simulink model "otwartaPetla"  (R2022b)
settings: Solver=VariableStepAuto  StartTime=0.0  StopTime=10.0  RelTol=1e-3
values from neighbouring files (symbols this model uses):
  pomoc = [1, 1, 1, 1]    [main.m]
  Y = [y, 0, 0, 0]'    [main.m]
settings Model: Creator=asialalala  LastModifiedBy=asialalala
settings DataIOCC: ReturnWorkspaceOutputs=off

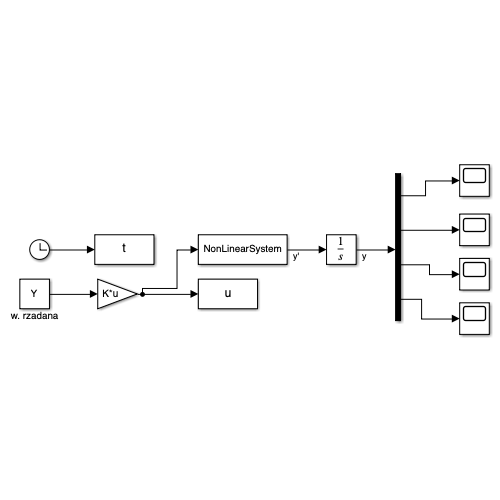
[thumbnail: Simulink's stored preview of the top-level diagram]
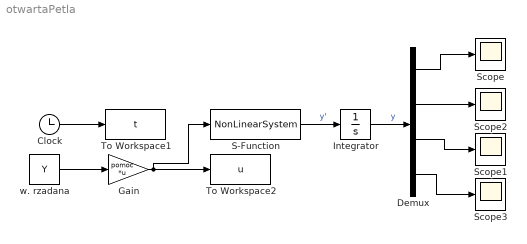
== system otwartaPetla ==
  Clock : Clock
  Demux : Demux
  Gain : Gain  Gain=pomoc  Multiplication=Matrix(K*u)
  Integrator : Integrator
  S-Function : S-Function  FunctionName=NonLinearSystem  Parameters=state0, params  SFunctionDeploymentMode=off  EnableBusSupport=off
  Scope{,1..3} (4 alike) : Scope
  To Workspace1 : ToWorkspace  VariableName=t  SampleTime=-1
  To Workspace2 : ToWorkspace  VariableName=u  SampleTime=-1
  w. rzadana : Constant  Value=Y
  wires:
  Demux/4 -> Scope3/1
  Demux/3 -> Scope1/1
  Demux/2 -> Scope2/1
  Gain/1 -> S-Function/1, To Workspace2/1
  S-Function/1 -> Integrator/1  "y'"
  Integrator/1 -> Demux/1  "y"
  Demux/1 -> Scope/1
  w. rzadana/1 -> Gain/1
  Clock/1 -> To Workspace1/1
